simulink model "kalmanfilterorjan"  (R2016b)
settings: Solver=FixedStepAuto  StartTime=0.0  StopTime=500  FixedStep=T  RelTol=1e-3
values from neighbouring files (symbols this model uses):
  Q = G'*G    [calc6.m]
  R = eye(8)    [FinInLLH.m]    (also in FinalSol.m; FinalSolV2.m; calc3sat.m = [1 0 0 0 0 0 0 0; calc4.m)
undefined symbols (not defined in the file or in its folder): A, A_d, B, B_d, d, g, H, k_d_phi, k_i_chi, k_i_phi, k_p_chi, k_p_phi, now, P_0, T, V_g
settings Model: Creator=Ørjan  LastModifiedBy=August

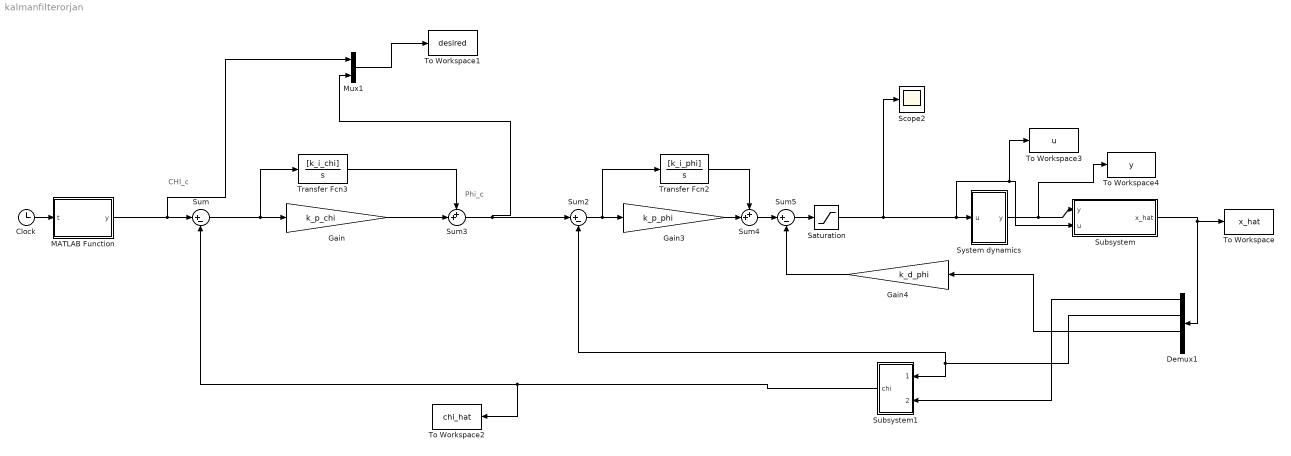
== system kalmanfilterorjan ==
  note: CHI_c
  note: Phi_c
  Clock : Clock
  Demux1 : Demux
  Gain : Gain  Gain=k_p_chi
  Gain3 : Gain  Gain=k_p_phi
  Gain4 : Gain  Gain=k_d_phi
  MATLAB Function : MATLAB Function  TreatAsAtomicUnit=on
  Mux1 : Mux  Inputs=2
  Saturation : Saturate  UpperLimit=25*pi/180  LowerLimit=-25*pi/180
  Scope2 : Scope
  Subsystem : Subsystem
  Subsystem1 : Subsystem
  Sum : Sum  Inputs=|+-
  Sum2 : Sum  Inputs=|+-
  Sum3 : Sum  Inputs=++|
  Sum4 : Sum  Inputs=++|
  Sum5 : Sum  Inputs=|+-
  System dynamics : Subsystem
  To Workspace : ToWorkspace  VariableName=x_hat  SaveFormat=Timeseries  SampleTime=-1
  To Workspace1 : ToWorkspace  VariableName=desired  SaveFormat=Timeseries  SampleTime=-1
  To Workspace2 : ToWorkspace  VariableName=chi_hat  SaveFormat=Timeseries  SampleTime=-1
  To Workspace3 : ToWorkspace  VariableName=u  SaveFormat=Timeseries  SampleTime=-1
  To Workspace4 : ToWorkspace  VariableName=y  SaveFormat=Timeseries  SampleTime=-1
  Transfer Fcn2 : TransferFcn  Numerator=[k_i_phi]  Denominator=[1 0]
  Transfer Fcn3 : TransferFcn  Numerator=[k_i_chi]  Denominator=[1 0]
  wires:
  Clock/1 -> MATLAB Function/1(t)
  MATLAB Function/1(y) -> Mux1/1, Sum/1
  Sum3/1 -> Mux1/2, Sum2/1
  Sum/1 -> Transfer Fcn3/1, Gain/1
  Gain/1 -> Sum3/2
  Transfer Fcn3/1 -> Sum3/1
  Sum2/1 -> Transfer Fcn2/1, Gain3/1
  Gain3/1 -> Sum4/2
  Transfer Fcn2/1 -> Sum4/1
  Gain4/1 -> Sum5/2
  Sum4/1 -> Sum5/1
  Sum5/1 -> Saturation/1
  Mux1/1 -> To Workspace1/1
  Saturation/1 -> Scope2/1, To Workspace3/1, Subsystem/2(u), System dynamics/1(u)
  System dynamics/1(y) -> To Workspace4/1, Subsystem/1(y)
  Subsystem/1(x_hat) -> Demux1/1, To Workspace/1
  Demux1/2 -> Subsystem1/1("phi "), Sum2/2
  Demux1/3 -> Gain4/1
  Subsystem1/1(chi) -> Sum/2, To Workspace2/1
  Demux1/1 -> Subsystem1/2(beta)

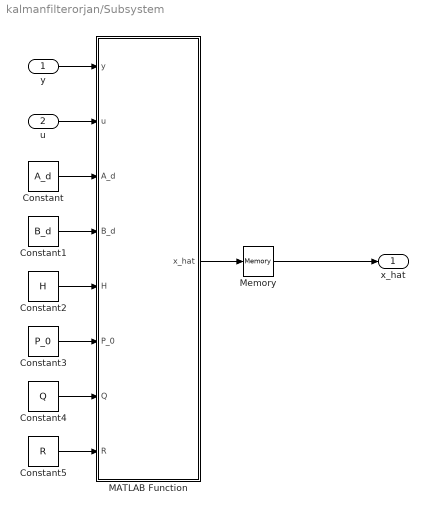
== system kalmanfilterorjan/Subsystem ==
  y : Inport
  u : Inport  Port=2
  Constant : Constant  Value=A_d
  Constant1 : Constant  Value=B_d
  Constant2 : Constant  Value=H
  Constant3 : Constant  Value=P_0
  Constant4 : Constant  Value=Q
  Constant5 : Constant  Value=R
  MATLAB Function : MATLAB Function  TreatAsAtomicUnit=on
  Memory : Memory  X0=[0 0 0 0]
  x_hat : Outport
  wires:
  MATLAB Function/1(x_hat) -> Memory/1
  y/1 -> MATLAB Function/1(y)
  u/1 -> MATLAB Function/2(u)
  Constant/1 -> MATLAB Function/3(A_d)
  Constant2/1 -> MATLAB Function/5(H)
  Constant3/1 -> MATLAB Function/6(P_0)
  Constant4/1 -> MATLAB Function/7(Q)
  Constant5/1 -> MATLAB Function/8(R)
  Constant1/1 -> MATLAB Function/4(B_d)
  Memory/1 -> x_hat/1

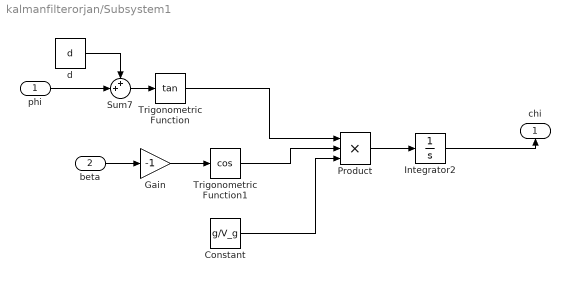
== system kalmanfilterorjan/Subsystem1 ==
  "phi " : Inport
  beta : Inport  Port=2
  Constant : Constant  Value=g/V_g
  Gain : Gain  Gain=-1
  Integrator2 : Integrator
  Product : Product  Inputs=3
  Sum7 : Sum  Inputs=++|
  Trigonometric Function : Trigonometry  Operator=tan
  Trigonometric Function1 : Trigonometry  Operator=cos
  d : Constant  Value=d
  chi : Outport
  wires:
  Gain/1 -> Trigonometric Function1/1
  Trigonometric Function/1 -> Product/1
  d/1 -> Sum7/1
  Product/1 -> Integrator2/1
  Trigonometric Function1/1 -> Product/2
  "phi "/1 -> Sum7/2
  Sum7/1 -> Trigonometric Function/1
  Integrator2/1 -> chi/1
  Constant/1 -> Product/3
  beta/1 -> Gain/1

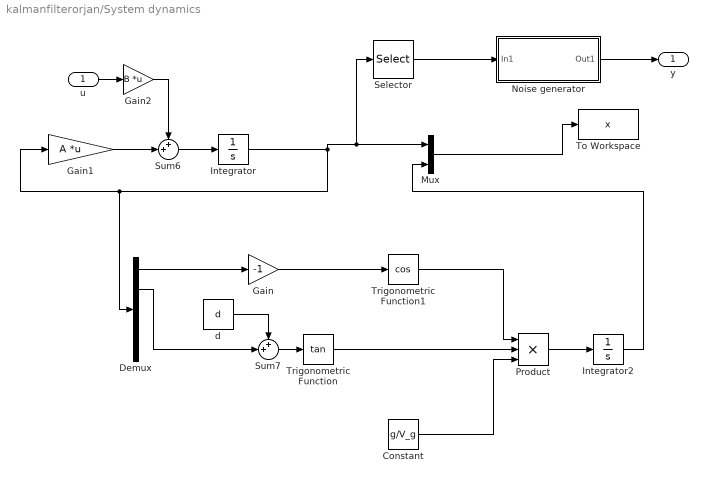
== system kalmanfilterorjan/System dynamics ==
  u : Inport
  Constant : Constant  Value=g/V_g
  Demux : Demux  Outputs=5
  Gain : Gain  Gain=-1
  Gain1 : Gain  Gain=A  Multiplication=Matrix(K*u)
  Gain2 : Gain  Gain=B  Multiplication=Matrix(K*u)
  Integrator : Integrator
  Integrator2 : Integrator
  Mux : Mux  Inputs=2
  Noise generator : Subsystem
  Product : Product  Inputs=3
  Selector : Selector  InputPortWidth=5  IndexOptions=Index vector (dialog)  Indices=[2 3 4]  OutputSizes=1
  Sum6 : Sum  Inputs=++|
  Sum7 : Sum  Inputs=++|
  To Workspace : ToWorkspace  VariableName=x  SaveFormat=Timeseries  SampleTime=-1
  Trigonometric Function : Trigonometry  Operator=tan
  Trigonometric Function1 : Trigonometry  Operator=cos
  d : Constant  Value=d
  y : Outport
  wires:
  Gain2/1 -> Sum6/1
  Demux/2 -> Sum7/2
  Sum6/1 -> Integrator/1
  Integrator/1 -> Selector/1, Mux/1, Demux/1, Gain1/1
  Gain1/1 -> Sum6/2
  Trigonometric Function/1 -> Product/2
  Integrator2/1 -> Mux/2
  Constant/1 -> Product/3
  Trigonometric Function1/1 -> Product/1
  Product/1 -> Integrator2/1
  Sum7/1 -> Trigonometric Function/1
  d/1 -> Sum7/1
  Mux/1 -> To Workspace/1
  Selector/1 -> Noise generator/1(In1)
  u/1 -> Gain2/1
  Noise generator/1(Out1) -> y/1
  Demux/1 -> Gain/1
  Gain/1 -> Trigonometric Function1/1

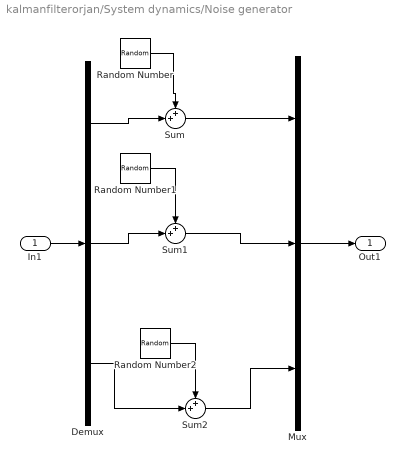
== system kalmanfilterorjan/System dynamics/Noise generator ==
  In1 : Inport
  Demux : Demux  Outputs=3
  Mux : Mux  Inputs=3
  Random Number : RandomNumber  Variance=0.0001  Seed=ceil(abs(5*round(abs(now*1e6 - fix(now*1e6))*1e5)))  SampleTime=T
  Random Number1 : RandomNumber  Variance=0.000008  Seed=ceil(abs(5*round(abs(now*1e6 - fix(now*1e6))*1e5)))  SampleTime=T
  Random Number2 : RandomNumber  Variance=0.000001  Seed=ceil(abs(5*round(abs(now*1e6 - fix(now*1e6))*1e5)))  SampleTime=T
  Sum : Sum  Inputs=++|
  Sum1 : Sum  Inputs=++|
  Sum2 : Sum  Inputs=++|
  Out1 : Outport
  wires:
  In1/1 -> Demux/1
  Mux/1 -> Out1/1
  Sum/1 -> Mux/1
  Demux/1 -> Sum/2
  Demux/2 -> Sum1/2
  Random Number1/1 -> Sum1/1
  Sum1/1 -> Mux/2
  Demux/3 -> Sum2/2
  Random Number2/1 -> Sum2/1
  Sum2/1 -> Mux/3
  Random Number/1 -> Sum/1

== matlab function kalmanfilterorjan/Subsystem/MATLAB Function ==
  data: y input; u input; x_hat output; A_d input; B_d input; H input; P_0 input; Q input; R input
function x_hat = fcn(y, u, A_d, B_d, H, P_0, Q, R)
persistent x_hat_old
persistent P;
if isempty(x_hat_old)
    x_hat_old = zeros(4, 1);
end
if isempty(P)
    P = P_0;
end
x_hat = A_d*x_hat_old + B_d*u;
P =A_d*P*A_d' + Q;


K = P*H'*inv(H*P*H'+R);
x_hat = x_hat + K*(y-H*x_hat);
P = (eye(4)-K*H)*P;

x_hat_old = x_hat;
end

== matlab function kalmanfilterorjan/MATLAB Function ==
  data: t input; y output
function y = fcn(t)
if t > 400
    u = -5;
elseif t > 300
    u = 10;
elseif t > 200
    u = 25;
elseif t > 100
    u = 10;
else
    u = 5;
end
y = u*pi/180;
